simulink model "outer_cycle"  (R2023a)
settings: Solver=VariableStepAuto  StartTime=0.0  StopTime=6  FixedStep=1e-3  RelTol=1e-3
libraries: simulink x4
settings Model: Creator=Gizem  LastModifiedBy=Gizem

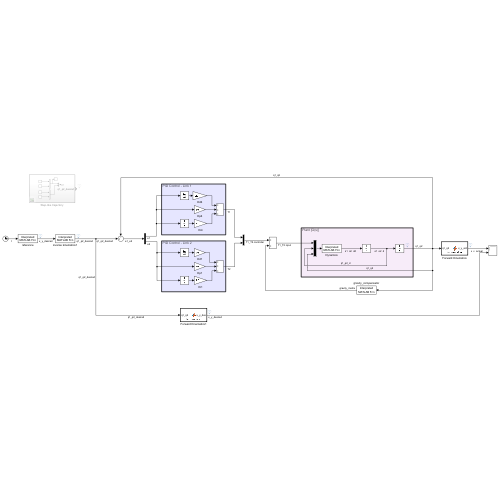
[thumbnail: Simulink's stored preview of the top-level diagram]
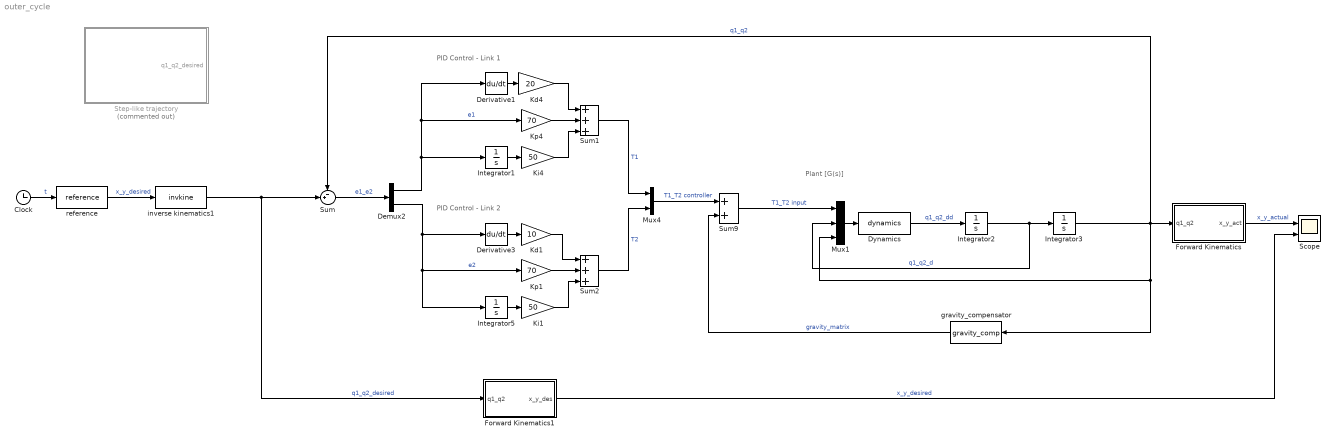
== system outer_cycle ==
  note: Plant [G(s)]
  note: PID Control - Link 2
  note: PID Control - Link 1
  Clock : Clock
  Demux2 : Demux  Outputs=2
  Derivative1 : Derivative
  Derivative3 : Derivative
  Dynamics : MATLABFcn  MATLABFcn=dynamics  OutputDimensions=2
  Forward Kinematics : MATLAB Function  TreatAsAtomicUnit=on
  Forward Kinematics1 : MATLAB Function  TreatAsAtomicUnit=on
  Integrator1 : Integrator
  Integrator2 : Integrator  InitialCondition=[0 0]
  Integrator3 : Integrator  InitialCondition=[0 0]
  Integrator5 : Integrator
  Kd1 : Gain  Gain=10
  Kd4 : Gain  Gain=20
  Ki1 : Gain  Gain=50
  Ki4 : Gain  Gain=50
  Kp1 : Gain  Gain=70
  Kp4 : Gain  Gain=70
  Mux1 : Mux  Inputs=3
  Mux4 : Mux  Inputs=2
  Scope : Scope  NumInputPorts=2
  Step-like trajectory : Subsystem  Commented=on
  Sum : Sum  Inputs=-+|
  Sum1 : Sum  Inputs=+++
  Sum2 : Sum  Inputs=+++
  Sum9 : Sum
  gravity_compensator : MATLABFcn  MATLABFcn=gravity_comp  OutputDimensions=2
  inverse kinematics1 : MATLABFcn  MATLABFcn=invkine  OutputDimensions=2
  reference : MATLABFcn  MATLABFcn=reference  OutputDimensions=2
  wires:
  Forward Kinematics1/1(x_y_des) -> Scope/2  "x_y_desired"
  Mux4/1 -> Sum9/1  "T1_T2 controller"
  Forward Kinematics/1(x_y_act) -> Scope/1  "x_y_actual"
  Sum9/1 -> Mux1/1  "T1_T2 input"
  Sum/1 -> Demux2/1  "e1_e2"
  Mux1/1 -> Dynamics/1
  Integrator2/1 -> Mux1/2, Integrator3/1  "q1_q2_d"
  Dynamics/1 -> Integrator2/1  "q1_q2_dd"
  Integrator3/1 -> Mux1/3, gravity_compensator/1, Forward Kinematics/1(q1_q2), Sum/1  "q1_q2"
  gravity_compensator/1 -> Sum9/2  "gravity_matrix"
  Demux2/1 -> Integrator1/1, Derivative1/1, Kp4/1  "e1"
  Kp4/1 -> Sum1/2
  Sum1/1 -> Mux4/1  "T1"
  Integrator1/1 -> Ki4/1
  Derivative1/1 -> Kd4/1
  Derivative3/1 -> Kd1/1
  Sum2/1 -> Mux4/2  "T2"
  Demux2/2 -> Integrator5/1, Kp1/1, Derivative3/1  "e2"
  Ki1/1 -> Sum2/3
  Ki4/1 -> Sum1/3
  Kp1/1 -> Sum2/2
  Kd1/1 -> Sum2/1
  Integrator5/1 -> Ki1/1
  Kd4/1 -> Sum1/1
  Clock/1 -> reference/1  "t"
  reference/1 -> inverse kinematics1/1  "x_y_desired"
  inverse kinematics1/1 -> Forward Kinematics1/1(q1_q2), Sum/2  "q1_q2_desired"

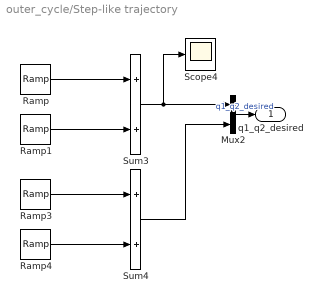
== system outer_cycle/Step-like trajectory ==
  Mux2 : Mux  Inputs=2
  Ramp : simulink/Sources/Ramp  slope=400  start=0  InitialOutput=0
  Ramp1 : simulink/Sources/Ramp  slope=-400  start=0.1  InitialOutput=0
  Ramp3 : simulink/Sources/Ramp  slope=400  start=0  InitialOutput=0
  Ramp4 : simulink/Sources/Ramp  slope=-400  start=0.1  InitialOutput=0
  Scope4 : Scope
  Sum3 : Sum
  Sum4 : Sum
  q1_q2_desired : Outport
  wires:
  Sum3/1 -> Scope4/1, Mux2/1
  Ramp1/1 -> Sum3/2
  Ramp3/1 -> Sum4/1
  Ramp4/1 -> Sum4/2
  Ramp/1 -> Sum3/1
  Sum4/1 -> Mux2/2
  Mux2/1 -> q1_q2_desired/1  "q1_q2_desired"

== matlab function outer_cycle/Forward Kinematics ==
  data: q1_q2 input; x_y_act output
function x_y_act = forwardkine(q1_q2)

% shaft to shaft length of the links
% link length 1 = 600mm = 0.6 m
% link length 2 = 400mm = 0.4 m

l1 = 0.6;
l2 = 0.4;

q1 = q1_q2(1);
q2 = q1_q2(2);

x1 = l1*cosd(q1);
y1 = l1*sind(q1);

x2 = x1 + l2*cosd(q1+q2);
y2 = y1 + l2*sind(q1+q2);
x_act = x2;
y_act = y2;

x_y_act = [x_act; y_act];
end

== matlab function outer_cycle/Forward Kinematics1 ==
  data: q1_q2 input; x_y_des output
function x_y_des = forwardkine(q1_q2)

% shaft to shaft length of the links
% link length 1 = 600mm = 0.6 m
% link length 2 = 400mm = 0.4 m

l1 = 0.6;
l2 = 0.4;

q1 = q1_q2(1);
q2 = q1_q2(2);

x1 = l1*cosd(q1);
y1 = l1*sind(q1);

x2 = x1 + l2*cosd(q1+q2);
y2 = y1 + l2*sind(q1+q2);
x_act = x2;
y_act = y2;

x_y_des = [x_act; y_act];
end
